simulink model "tx2rx_link_simulink"  (R2022a)
settings: Solver=VariableStepAuto  StartTime=0.0  StopTime=simParam.time  RelTol=1e-3
undefined symbols (not defined in the file or in its folder): simParam
libraries: simrfV2util1 x6, simrfV2sources1 x3, simrfV2elements x2
settings Model: Creator=zg88  LastModifiedBy=zg88

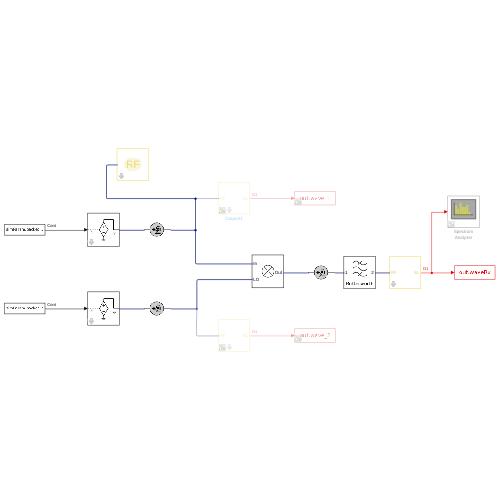
[thumbnail: Simulink's stored preview of the top-level diagram]
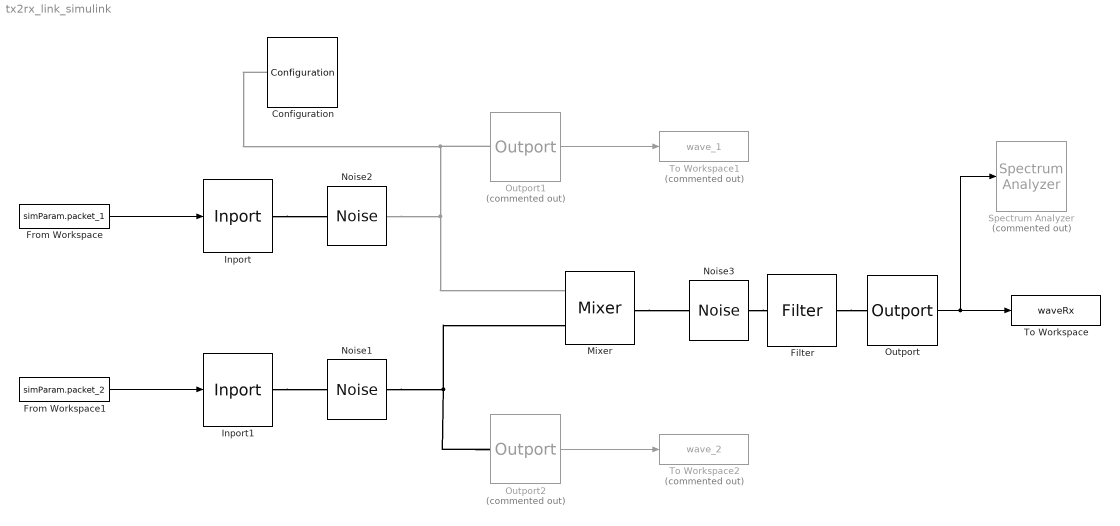
== system tx2rx_link_simulink ==
  Configuration : simrfV2util1/Configuration  AutoFreq=on  Tones="[1         1.5] GHz"  Harmonics="[5  5]"  NormalizeCarrierPower=on  SolverType=Auto  UseCCode=on  StepSize=1 / simParam.analog s  AddNoise=on  defaultRNG=on  Seed=0  Temperature=simParam.temperature K  SolverDelFlag=0  AbsTol=1e-6  RelTol=1e-3  MaxIter=10  ErrorEstimationType=2-norm over all variables  EnableInterpFilter=on  HiddenFIRfilterControllerParam=off  SmallSignalApprox=off  AllSimFreqs=on  SimFreqs=[] Hz  SimFreqsInternal=[]  SamplesPerFrame=1
      settings: SourceProductBaseCode=RB
  Filter : simrfV2elements/Filter  classname=filter  DesignMethod=Butterworth  ResponseType=Bandpass  Implementation=LC Tee  ImplementationIdeal=Constant per carrier  ImplementationRational=Transfer function  UseFilterOrder=on  FilterOrder=8  PassFreq_lp=1000000 Hz  PassFreq_hp=2 GHz  PassFreq_bp=[simParam.passLow simParam.passHigh] Hz  PassFreq_bs=[1 4] GHz  PassAtten=1  StopFreq_lp=2 GHz  StopFreq_hp=1 GHz  StopFreq_bp=[1.5 3.5] GHz  StopFreq_bs=[2.1 2.9] GHz  StopAtten=40  Rsrc=50  Rload=50  AutoImpulseLength=on  ImpulseLength=1e-10 s  InternalGrounding=on  PlotFuncLeft=Voltage transfer  PlotLeftForm=Magnitude (decibels)  PlotRightOnVT=None  PlotRightNoTD=None  PlotRightNoGD=None  PlotRightNoIR=None  PlotRightNoSR=None  PlotRightForm=Magnitude (decibels)  FreqPoints=logspace(0,10,101)  Freq_unit=Hz  TimePoints=linspace(0,1,1e6+1)  Time_unit=s  XaxisScale=Linear  YaxisScale=Linear  needRedraw=0
      settings: SourceProductBaseCode=RB
  From Workspace : FromWorkspace  VariableName=simParam.packet_1
  From Workspace1 : FromWorkspace  VariableName=simParam.packet_2
  Inport : simrfV2util1/Inport  SimulinkInputSignalType=Ideal voltage  CarrierFreq=simParam.carrier_1 Hz  ZS=0  InternalGrounding=on
      settings: SourceProductBaseCode=RB
  Inport1 : simrfV2util1/Inport  SimulinkInputSignalType=Ideal voltage  CarrierFreq=simParam.carrier_2 Hz  ZS=0  InternalGrounding=on
      settings: SourceProductBaseCode=RB
  Mixer : simrfV2elements/Mixer  classname=mixer  Source_linear_gain=Available power gain  linear_gain=0 dB  Zin=50  Zout=50  ZLO=inf  Source_Poly=Even and odd order  Poly_Coeffs=[0 1]  IPType=Output  IP2=Inf dBm  IP3=Inf dBm  P1dB=Inf dBm  Psat=Inf dBm  Gcomp=Inf dBm  NF=0  InternalGrounding=on
      settings: SourceProductBaseCode=RB
  Noise1 : simrfV2sources1/Noise  SimulinkInputSignalType=Ideal voltage  NoiseType=White  NoisePSD=simParam.noiseIn*50  CarrierFreq=0 Hz  AutoImpulseLength=on  ImpulseLength=1e-10 s  InternalGrounding=off
      settings: SourceProductBaseCode=RB
  Noise2 : simrfV2sources1/Noise  SimulinkInputSignalType=Ideal voltage  NoiseType=White  NoisePSD=simParam.noiseIn*50  CarrierFreq=0 Hz  AutoImpulseLength=on  ImpulseLength=1e-10 s  InternalGrounding=off
      settings: SourceProductBaseCode=RB
  Noise3 : simrfV2sources1/Noise  SimulinkInputSignalType=Ideal voltage  NoiseType=White  NoisePSD=simParam.noiseOut*50  CarrierFreq=0 Hz  AutoImpulseLength=on  ImpulseLength=1e-10 s  InternalGrounding=off
      settings: SourceProductBaseCode=RB
  Outport : simrfV2util1/Outport  SensorType=Ideal voltage  OutputFormat=Complex Baseband  CarrierFreq=simParam.carrierRx Hz  ZL=Inf  InternalGrounding=on  StepSize=1e-6 s  AutoStep=on
      settings: SourceProductBaseCode=RB
  Outport1 : simrfV2util1/Outport  Commented=on  SensorType=Ideal voltage  OutputFormat=Complex Baseband  CarrierFreq=simParam.carrier_1 Hz  ZL=Inf  InternalGrounding=on  StepSize=1e-6 s  AutoStep=on
      settings: SourceProductBaseCode=RB
  Outport2 : simrfV2util1/Outport  Commented=on  SensorType=Ideal voltage  OutputFormat=Complex Baseband  CarrierFreq=simParam.carrier_2 Hz  ZL=Inf  InternalGrounding=on  StepSize=1e-6 s  AutoStep=on
      settings: SourceProductBaseCode=RB
  Spectrum Analyzer : SpectrumAnalyzer  Tag=simrfV2util1/Spectrum Analyzer  Commented=on
  To Workspace : ToWorkspace  VariableName=waveRx  SaveFormat=Timeseries  SampleTime=-1
  To Workspace1 : ToWorkspace  Commented=on  VariableName=wave_1  SaveFormat=Timeseries  SampleTime=-1
  To Workspace2 : ToWorkspace  Commented=on  VariableName=wave_2  SaveFormat=Timeseries  SampleTime=-1
  wires:
  From Workspace/1 -> Inport/1
  From Workspace1/1 -> Inport1/1
  Outport1/1 -> To Workspace1/1
  Outport2/1 -> To Workspace2/1
  Outport/1 -> Spectrum Analyzer/1, To Workspace/1
  connections:
  Outport1/LConn1 -- Noise2/RConn1 -- Mixer/LConn1 -- Configuration/LConn1
  Inport1/RConn1 -- Noise1/LConn1
  Filter/RConn1 -- Outport/LConn1
  Noise1/RConn1 -- Outport2/LConn1 -- Mixer/LConn2
  Inport/RConn1 -- Noise2/LConn1
  Mixer/RConn1 -- Noise3/LConn1
  Noise3/RConn1 -- Filter/LConn1
